simulink model "Vehicle_Powertrain_01"  (R2014a)
settings: Solver=ode45  StartTime=0.0  StopTime=10  RelTol=1e-3
libraries: fl_lib x3, sdl_lib x2, nesl_utility x1
Description:
  | Copyright 2014 The MathWorks, Inc.
settings Model: Creator=smiller  LastModifiedBy=smiller
settings DataIOCC: SignalLoggingSaveFormat=ModelDataLogs
settings OptimizationCC: ExpressionDepthLimit=2147483647
settings DebuggingCC: UnderspecifiedInitializationDetection=Classic  FcnCallInpInsideContextMsg=UseLocalSettings  StateNameClashWarn=warning
settings GRTTargetCC: CombineOutputUpdateFcns=off  GRTInterface=on

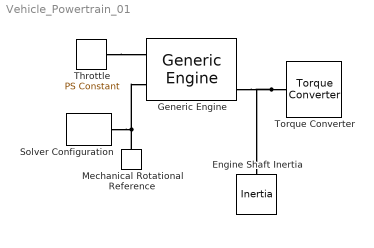
== system Vehicle_Powertrain_01 ==
  Engine Shaft Inertia : fl_lib/Mechanical/Rotational Elements/Inertia  inertia=0.2 kg*m^2  w_specify=on  w_priority=High  w=800 rpm  t_specify=off  t_priority=High  t=0 N*m
  Generic Engine : sdl_lib/Engines/Generic Engine  model_parameterization=1  engine_type=1  P_max=1.5e+5 W  w_P_max=4.5e+3 rpm  w_max=6e+3 rpm  w_min=500 rpm  w_tab=[ 500 1000 2e+3 3e+3 4e+3 5e+3 6e+3 7e+3 ] rpm  trq_tab=[ 380 380 380 380 350 280 200 80 ] N*m  pwr_tab=[ 2e+4 4e+4 7.8e+4 1.2e+5 1.45e+5 1.48e+5 1.25e+5 6e+4 ] W  interp_method=1  model_inertia=0  inertia=1 kg*m^2  initial_velocity=800 rpm  model_time_constant=0  time_constant=0.2 s  T0=0  w_thr=100 rpm  idle_speed=0  idle_speed_reference=1000 rpm  tau_controller=1 s  idle_w_thr=1 rpm  fc_model=1  fc_per_rev=25 mg/rev  displaced_volume=400 cm^3  rev_per_cycle=2  fc_w_tab=[ 1000 2e+3 3e+3 4e+3 5e+3 6e+3 ] rpm  fc_trq_tab=[ 0 80 160 200 240 320 360 400 ] N*m  fc_tab=[ 0.5 0.9 1.4 1.6 1.9 2.7 3.4 4.4; 1 1.7 2.7 3.1 3.6 5 6 7.4; 1.4 2.7 4 4.8 5.6 7.5 8.5 10.5; 2 3.6 5.8 6.7 8 10.4 11.7 13.3; 2.5 4.8 7.9 9.4 10.8 14 16.2 18.6; 3.1 6 10.3 11.9 13.8 18.4 22 26.5 ] g/s  bmep_tab=[ 0 250 500 625 750 1000 1.15e+3 1.25e+3 ] kPa  bsfc_tab=[ 410 380 300 280 270 290 320 380; 410 370 290 270 260 270 285 320; 415 380 290 275 265 270 270 300; 420 390 310 290 285 280 280 285; 430 410 340 320 310 300 310 320; 450 430 370 340 330 330 350 380 ] g/hr/kW  fc_interp_method=1
  Mechanical Rotational Reference : fl_lib/Mechanical/Rotational Elements/Mechanical Rotational Reference
  Solver Configuration : nesl_utility/Solver Configuration  PhysicalDomain=network_engine_domain  SubClassName=solver  LeftPortType=input  RightPortType=generic  Accelerate=off  Tones=[]  Harmonics=[]  SimulateNoise=off  Profile=off  UseLocalSampling=off  EnableSwitchedLinearOptims=on  FrequencyDomain=off  UseCCode=off  RelTol=0.001  AbsTol=1e-06  MinStep=1e-09  ToWorkspace=off  DoDC=off  ResidualTolerance=1e-9  UseLocalSolver=off  LocalSolverChoice=NE_BACKWARD_EULER_ADVANCER  LocalSolverSampleTime=.001  DoFixedCost=off  MaxNonlinIter=3  MaxModeIter=2  LinearAlgebra=Sparse  DelaysMemoryBudget=1024  AutomaticFiltering=on  FilteringTimeConstant=0.001
  Throttle : fl_lib/Physical Signals/Sources/PS Constant  constant=0.5
  Torque Converter : sdl_lib/Couplings & Drives/Torque Converter  n_vector=[ 0 0.5 0.6 0.7 0.8 0.81 0.82 0.83 0.84 0.85 0.86 0.87 0.88 0.89 0.9 0.92 0.94 0.96 0.97 ]  trq_vector=[ 2.232 1.5462 1.4058 1.2746 1.1528 1.1412 1.1296 1.1181 1.1067 1.0955 1.0843 1.0732 1.0622 1.0513 1.0405 1.0192 0.9983 0.9983 0.9983 ]  cf_vector_parameterization=1  cf_vector_reference_speed=1  cf_vector=[ 12.2938 12.8588 13.1452 13.6285 14.6163 14.7747 14.9516 15.1502 15.3748 15.6309 15.9253 16.2675 16.6698 17.1492 17.7298 19.3503 22.1046 29.9986 50 ] (rad/s)/(N*m)^0.5  cf_vector_sq=[ 0.006615999999999999 0.006048 0.005787 0.005384 0.004681 0.004581 0.004473 0.004357 0.00423 0.004093 0.003943 0.003779 0.003599 0.0034 0.003181 0.002671 0.002047 0.001111 4e-4 ] N*m/(rad/s)^2  interp_method=1  extrap_method=1  model_lag=0  tau=0.02 s  initial_trq_ratio=0
  connections:
  Mechanical Rotational Reference/LConn1 -- Generic Engine/LConn2 -- Solver Configuration/RConn1
  Throttle/RConn1 -- Generic Engine/LConn1
  Torque Converter/LConn1 -- Generic Engine/RConn3 -- Engine Shaft Inertia/LConn1
